simulink model "TwoArea_MA_FixedWM"  (R2020b)
settings: Solver=ode3  StartTime=0.0  StopTime=t  FixedStep=0.01  RelTol=1e-3
values from neighbouring files (symbols this model uses):
  AGC_midway = 0    [TwoAreaAGC_Parameters_Start_MA.m]    (also in result_agcimprovement.m = 1; result_replayimpact.m; result_replayimpactvaryingload.m; result_replaywithoutwm.m)
  Apc = [-par.D/(2*par.H)  1/(2*par.H)  0  -1/(2*par.H) ... (first row only)    [get_ssplant_1turb.m]
  Aq = zeros(N,N,nyp)    [offline_watermarking.m]
  attack_cont = 1    [TwoAreaAGC_Parameters_Start_MA.m]    (also in result_agcimprovement.m = 0; result_replayimpact.m; result_replayimpactvaryingload.m = 0; result_replaywithoutwm.m)
  attack_meas = 1    [TwoAreaAGC_Parameters_Start_MA.m]    (also in result_agcimprovement.m = 0; result_replayimpact.m; result_replayimpactvaryingload.m; result_replaywithoutwm.m)
  attack_start = 300    [TwoAreaAGC_Parameters_Start_MA.m]
  attack_type = 1    [TwoAreaAGC_Parameters_Start_MA.m]    (also in result_agcimprovement.m; result_replayimpact.m; result_replayimpactvaryingload.m; result_replaywithoutwm.m)
  Aw = zeros(N,N,nyp)    [offline_watermarking.m]
  Bpc = [0  -1/(2*par.H) ... (first row only)    [get_ssplant_1turb.m]
  Bq = zeros(N,1,nyp)    [offline_watermarking.m]
  Bw = zeros(N,1,nyp)    [offline_watermarking.m]
  C_sysd = c2d(C_sysc,ts_c)    [get_sscontr_2area.m]
  Cpc = [1 0 0 0 ... (first row only)    [get_ssplant_1turb.m]
  Cq = zeros(1,N,nyp)    [offline_watermarking.m]
  Cw = zeros(1,N,nyp)    [offline_watermarking.m]
  Dq = zeros(1,1,nyp)    [offline_watermarking.m]
  Dw = zeros(1,1,nyp)    [offline_watermarking.m]
  Ps = 2    [TwoAreaAGC_Parameters_Start_MA.m]
  scaling_replay = 2    [TwoAreaAGC_Parameters_Start_MA.m]    (also in result_agcimprovement.m = 1; result_replayimpact.m; result_replayimpactvaryingload.m; result_replaywithoutwm.m)
  status_load = 0    [TwoAreaAGC_Parameters_Start_MA.m]    (also in result_agcimprovement.m; result_replayimpact.m; result_replayimpactvaryingload.m = 1; result_replaywithoutwm.m)
  status_wm = 1    [TwoAreaAGC_Parameters_Start_MA.m]    (also in result_agcimprovement.m = 0; result_replayimpact.m = 0; result_replayimpactvaryingload.m = 0; result_replaywithoutwm.m = 0)
  ts = 1e-2    (= 0.01)    [TwoAreaAGC_Parameters_Start_MA.m]
undefined symbols (not defined in the file or in its folder): Ag, Ah, Bg, Bh, ca, Cg, Ch, Dg, Dh, DiscIntNeverNeededParam, Dpc, eta1, eta2, L1, L2, obs1, obs2, P1_sysd, P2_sysd, par1, par2, wm, xi1, xi2
libraries: cstblocks x16, dspsrcs4 x5, eeLuenbergerObserver x2
(part 2 of 2)

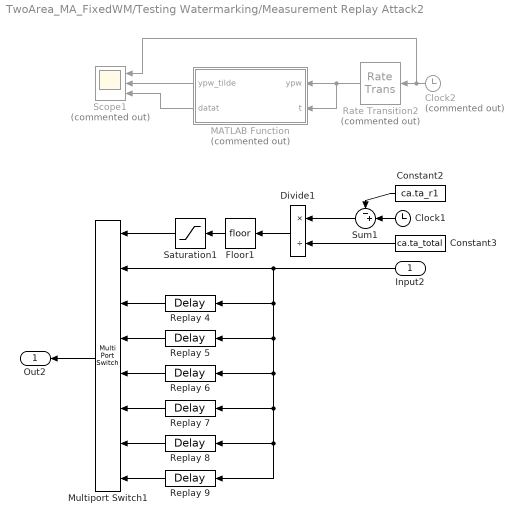
== system TwoArea_MA_FixedWM/Testing Watermarking/Measurement Replay Attack2 ==
  Input2 : Inport
  Clock1 : Clock
  Clock2 : Clock  Commented=on
  Constant2 : Constant  Value=ca.ta_r1
  Constant3 : Constant  Value=ca.ta_total
  Divide1 : Product  Inputs=*/  OutMin=0  OutMax=3  SaturateOnIntegerOverflow=on
  Floor1 : Rounding
  MATLAB Function : MATLAB Function  Commented=on  TreatAsAtomicUnit=on
  Multiport Switch1 : MultiPortSwitch  DataPortOrder=Zero-based contiguous  Inputs=7  zeroidx=on
  Rate Transition2 : RateTransition  Commented=on  OutPortSampleTime=1
  Replay 4 : TransportDelay  DelayTime=ca.ta_total
  Replay 5 : TransportDelay  DelayTime=ca.ta_total*2
  Replay 6 : TransportDelay  DelayTime=ca.ta_total*3
  Replay 7 : TransportDelay  DelayTime=ca.ta_total*4
  Replay 8 : TransportDelay  DelayTime=ca.ta_total*5
  Replay 9 : TransportDelay  DelayTime=ca.ta_total*6
  Saturation1 : Saturate  UpperLimit=6  LowerLimit=0
  Scope1 : Scope  Commented=on  NumInputPorts=3
  Sum1 : Sum  Inputs=-+|
  Out2 : Outport
  wires:
  MATLAB Function/1(ypw_tilde) -> Scope1/2
  MATLAB Function/2(datat) -> Scope1/3
  Rate Transition2/1 -> MATLAB Function/2(t), MATLAB Function/1(ypw)
  Clock2/1 -> Scope1/1, Rate Transition2/1
  Saturation1/1 -> Multiport Switch1/1
  Input2/1 -> Replay 9/1, Replay 8/1, Replay 7/1, Replay 6/1, Replay 5/1, Replay 4/1, Multiport Switch1/2
  Sum1/1 -> Divide1/1
  Replay 4/1 -> Multiport Switch1/3
  Floor1/1 -> Saturation1/1
  Replay 5/1 -> Multiport Switch1/4
  Multiport Switch1/1 -> Out2/1
  Constant3/1 -> Divide1/2
  Replay 9/1 -> Multiport Switch1/8
  Replay 8/1 -> Multiport Switch1/7
  Divide1/1 -> Floor1/1
  Replay 7/1 -> Multiport Switch1/6
  Constant2/1 -> Sum1/1
  Clock1/1 -> Sum1/2
  Replay 6/1 -> Multiport Switch1/5

== system TwoArea_MA_FixedWM/W (Watermarker)/ W selector2 ==
  Constant10 : Constant  Value=Bw  VectorParams1D=off
  Constant11 : Constant  Value=Cw  VectorParams1D=off
  Constant12 : Constant  Value=Dw  VectorParams1D=off
  Constant9 : Constant  Value=Aw  VectorParams1D=off
  Counter : Subsystem
  MATLAB Function : MATLAB Function  TreatAsAtomicUnit=on
  Aw : Outport
  Bw : Outport  Port=2
  Cw : Outport  Port=3
  Dw : Outport  Port=4
  wires:
  Constant9/1 -> MATLAB Function/2(Aa)
  Constant10/1 -> MATLAB Function/3(Ba)
  Constant11/1 -> MATLAB Function/4(Ca)
  Constant12/1 -> MATLAB Function/5(Da)
  Counter/1(WM_rotation) -> MATLAB Function/1(WM_rotation)
  MATLAB Function/4(D) -> Dw/1
  MATLAB Function/3(C) -> Cw/1
  MATLAB Function/2(B) -> Bw/1
  MATLAB Function/1(A) -> Aw/1

== system TwoArea_MA_FixedWM/W (Watermarker)/W selector 1 ==
  Constant10 : Constant  Value=Bw  VectorParams1D=off
  Constant11 : Constant  Value=Cw  VectorParams1D=off
  Constant12 : Constant  Value=Dw  VectorParams1D=off
  Constant9 : Constant  Value=Aw  VectorParams1D=off
  Counter : Subsystem
  MATLAB Function : MATLAB Function  TreatAsAtomicUnit=on
  Aw : Outport
  Bw : Outport  Port=2
  Cw : Outport  Port=3
  Dw : Outport  Port=4
  wires:
  Constant9/1 -> MATLAB Function/2(Aa)
  Constant10/1 -> MATLAB Function/3(Ba)
  Constant11/1 -> MATLAB Function/4(Ca)
  Constant12/1 -> MATLAB Function/5(Da)
  Counter/1(WM_rotation) -> MATLAB Function/1(WM_rotation)
  MATLAB Function/4(D) -> Dw/1
  MATLAB Function/3(C) -> Cw/1
  MATLAB Function/2(B) -> Bw/1
  MATLAB Function/1(A) -> Aw/1

== system TwoArea_MA_FixedWM/W (Watermarker)/W selector3 ==
  Constant10 : Constant  Value=Bw  VectorParams1D=off
  Constant11 : Constant  Value=Cw  VectorParams1D=off
  Constant12 : Constant  Value=Dw  VectorParams1D=off
  Constant9 : Constant  Value=Aw  VectorParams1D=off
  Counter : Subsystem
  MATLAB Function : MATLAB Function  TreatAsAtomicUnit=on
  Aw : Outport
  Bw : Outport  Port=2
  Cw : Outport  Port=3
  Dw : Outport  Port=4
  wires:
  Constant9/1 -> MATLAB Function/2(Aa)
  Constant10/1 -> MATLAB Function/3(Ba)
  Constant11/1 -> MATLAB Function/4(Ca)
  Constant12/1 -> MATLAB Function/5(Da)
  Counter/1(WM_rotation) -> MATLAB Function/1(WM_rotation)
  MATLAB Function/4(D) -> Dw/1
  MATLAB Function/3(C) -> Cw/1
  MATLAB Function/2(B) -> Bw/1
  MATLAB Function/1(A) -> Aw/1

== system TwoArea_MA_FixedWM/G (Watermarker)/ G selector/Counter ==
  Constant34 : Constant
  Constant35 : Constant
  Delay : Delay  DelayLength=1  SampleTime=wm.t
  Sum : Sum
  Switch : Switch  Criteria=u2 > Threshold  Threshold=3
  WM_rotation : Outport
  wires:
  Constant35/1 -> Switch/1
  Constant34/1 -> Sum/1
  Delay/1 -> Switch/2, Sum/2
  Sum/1 -> Switch/3
  Switch/1 -> WM_rotation/1, Delay/1

== system TwoArea_MA_FixedWM/G (Watermarker)/ G selector1/Counter ==
  Constant34 : Constant
  Constant35 : Constant
  Delay : Delay  DelayLength=1  SampleTime=wm.t
  Sum : Sum
  Switch : Switch  Criteria=u2 > Threshold  Threshold=3
  WM_rotation : Outport
  wires:
  Constant35/1 -> Switch/1
  Constant34/1 -> Sum/1
  Delay/1 -> Switch/2, Sum/2
  Sum/1 -> Switch/3
  Switch/1 -> WM_rotation/1, Delay/1

== system TwoArea_MA_FixedWM/H (Watermark Remover)/ H selector/Counter ==
  Constant34 : Constant
  Constant35 : Constant
  Delay : Delay  DelayLength=1  SampleTime=wm.t
  Sum : Sum
  Switch : Switch  Criteria=u2 > Threshold  Threshold=3
  WM_rotation : Outport
  wires:
  Constant35/1 -> Switch/1
  Constant34/1 -> Sum/1
  Delay/1 -> Switch/2, Sum/2
  Sum/1 -> Switch/3
  Switch/1 -> WM_rotation/1, Delay/1

== system TwoArea_MA_FixedWM/H (Watermark Remover)/ H selector1/Counter ==
  Constant34 : Constant
  Constant35 : Constant
  Delay : Delay  DelayLength=1  SampleTime=wm.t
  Sum : Sum
  Switch : Switch  Criteria=u2 > Threshold  Threshold=3
  WM_rotation : Outport
  wires:
  Constant35/1 -> Switch/1
  Constant34/1 -> Sum/1
  Delay/1 -> Switch/2, Sum/2
  Sum/1 -> Switch/3
  Switch/1 -> WM_rotation/1, Delay/1

== system TwoArea_MA_FixedWM/Q (Watermark Remover)/ Q selector/Counter ==
  Constant34 : Constant
  Constant35 : Constant
  Delay : Delay  DelayLength=1  SampleTime=wm.t
  Sum : Sum
  Switch : Switch  Criteria=u2 > Threshold  Threshold=3
  WM_rotation : Outport
  wires:
  Constant35/1 -> Switch/1
  Constant34/1 -> Sum/1
  Delay/1 -> Switch/2, Sum/2
  Sum/1 -> Switch/3
  Switch/1 -> WM_rotation/1, Delay/1

== system TwoArea_MA_FixedWM/Q (Watermark Remover)/ Q selector1/Counter ==
  Constant34 : Constant
  Constant35 : Constant
  Delay : Delay  DelayLength=1  SampleTime=wm.t
  Sum : Sum
  Switch : Switch  Criteria=u2 > Threshold  Threshold=3
  WM_rotation : Outport
  wires:
  Constant35/1 -> Switch/1
  Constant34/1 -> Sum/1
  Delay/1 -> Switch/2, Sum/2
  Sum/1 -> Switch/3
  Switch/1 -> WM_rotation/1, Delay/1

== system TwoArea_MA_FixedWM/Q (Watermark Remover)/ Q selector2/Counter ==
  Constant34 : Constant
  Constant35 : Constant
  Delay : Delay  DelayLength=1  SampleTime=wm.t
  Sum : Sum
  Switch : Switch  Criteria=u2 > Threshold  Threshold=3
  WM_rotation : Outport
  wires:
  Constant35/1 -> Switch/1
  Constant34/1 -> Sum/1
  Delay/1 -> Switch/2, Sum/2
  Sum/1 -> Switch/3
  Switch/1 -> WM_rotation/1, Delay/1

== system TwoArea_MA_FixedWM/Testing Watermarking/ G selector/Counter ==
  Constant34 : Constant
  Constant35 : Constant
  Delay : Delay  DelayLength=1  SampleTime=wm.t
  Sum : Sum
  Switch : Switch  Criteria=u2 > Threshold  Threshold=3
  WM_rotation : Outport
  wires:
  Constant35/1 -> Switch/1
  Constant34/1 -> Sum/1
  Delay/1 -> Switch/2, Sum/2
  Sum/1 -> Switch/3
  Switch/1 -> WM_rotation/1, Delay/1

== system TwoArea_MA_FixedWM/Testing Watermarking/ H selector/Counter ==
  Constant34 : Constant
  Constant35 : Constant
  Delay : Delay  DelayLength=1  SampleTime=wm.t
  Sum : Sum
  Switch : Switch  Criteria=u2 > Threshold  Threshold=3
  WM_rotation : Outport
  wires:
  Constant35/1 -> Switch/1
  Constant34/1 -> Sum/1
  Delay/1 -> Switch/2, Sum/2
  Sum/1 -> Switch/3
  Switch/1 -> WM_rotation/1, Delay/1

== system TwoArea_MA_FixedWM/Testing Watermarking/ Q selector/Counter ==
  Constant34 : Constant
  Constant35 : Constant
  Delay : Delay  DelayLength=1  SampleTime=wm.t
  Sum : Sum
  Switch : Switch  Criteria=u2 > Threshold  Threshold=3
  WM_rotation : Outport
  wires:
  Constant35/1 -> Switch/1
  Constant34/1 -> Sum/1
  Delay/1 -> Switch/2, Sum/2
  Sum/1 -> Switch/3
  Switch/1 -> WM_rotation/1, Delay/1

== system TwoArea_MA_FixedWM/Testing Watermarking/ W selector/Counter ==
  Constant34 : Constant
  Constant35 : Constant
  Delay : Delay  DelayLength=1  SampleTime=wm.t
  Sum : Sum
  Switch : Switch  Criteria=u2 > Threshold  Threshold=3
  WM_rotation : Outport
  wires:
  Constant35/1 -> Switch/1
  Constant34/1 -> Sum/1
  Delay/1 -> Switch/2, Sum/2
  Sum/1 -> Switch/3
  Switch/1 -> WM_rotation/1, Delay/1

== system TwoArea_MA_FixedWM/W (Watermarker)/ W selector2/Counter ==
  Constant34 : Constant
  Constant35 : Constant
  Delay : Delay  DelayLength=1  SampleTime=wm.t
  Sum : Sum
  Switch : Switch  Criteria=u2 > Threshold  Threshold=3
  WM_rotation : Outport
  wires:
  Constant35/1 -> Switch/1
  Constant34/1 -> Sum/1
  Delay/1 -> Switch/2, Sum/2
  Sum/1 -> Switch/3
  Switch/1 -> WM_rotation/1, Delay/1

== system TwoArea_MA_FixedWM/W (Watermarker)/W selector 1/Counter ==
  Constant34 : Constant
  Constant35 : Constant
  Delay : Delay  DelayLength=1  SampleTime=wm.t
  Sum : Sum
  Switch : Switch  Criteria=u2 > Threshold  Threshold=3
  WM_rotation : Outport
  wires:
  Constant35/1 -> Switch/1
  Constant34/1 -> Sum/1
  Delay/1 -> Switch/2, Sum/2
  Sum/1 -> Switch/3
  Switch/1 -> WM_rotation/1, Delay/1

== system TwoArea_MA_FixedWM/W (Watermarker)/W selector3/Counter ==
  Constant34 : Constant
  Constant35 : Constant
  Delay : Delay  DelayLength=1  SampleTime=wm.t
  Sum : Sum
  Switch : Switch  Criteria=u2 > Threshold  Threshold=3
  WM_rotation : Outport
  wires:
  Constant35/1 -> Switch/1
  Constant34/1 -> Sum/1
  Delay/1 -> Switch/2, Sum/2
  Sum/1 -> Switch/3
  Switch/1 -> WM_rotation/1, Delay/1

== matlab function TwoArea_MA_FixedWM/W (Watermarker)/ W selector2/MATLAB Function ==
  data: WM_rotation input; A output; Aa input; Ba input; Ca input; Da input; B output; C output; D output
function [A,B,C,D] = WM_Selector(WM_rotation,Aa,Ba,Ca,Da)
% Select the correct watermark state space matrices for the current time
A = Aa(:,:,WM_rotation);
B = Ba(:,:,WM_rotation);
C = Ca(:,:,WM_rotation);
D = Da(:,:,WM_rotation);

== matlab function TwoArea_MA_FixedWM/W (Watermarker)/W selector 1/MATLAB Function ==
  data: WM_rotation input; A output; Aa input; Ba input; Ca input; Da input; B output; C output; D output
function [A,B,C,D] = WM_Selector(WM_rotation,Aa,Ba,Ca,Da)
% Select the correct watermark state space matrices for the current time
A = Aa(:,:,WM_rotation);
B = Ba(:,:,WM_rotation);
C = Ca(:,:,WM_rotation);
D = Da(:,:,WM_rotation);

== matlab function TwoArea_MA_FixedWM/Testing Watermarking/ H selector/MATLAB Function ==
  data: WM_rotation input; A output; Aa input; Ba input; Ca input; Da input; B output; C output; D output
function [A,B,C,D] = WM_Selector(WM_rotation,Aa,Ba,Ca,Da)
% Select the correct watermark state space matrices for the current time
A = Aa(:,:,WM_rotation);
B = Ba(:,:,WM_rotation);
C = Ca(:,:,WM_rotation);
D = Da(:,:,WM_rotation);

== matlab function TwoArea_MA_FixedWM/Testing Watermarking/ G selector/MATLAB Function ==
  data: WM_rotation input; A output; Aa input; Ba input; Ca input; Da input; B output; C output; D output
function [A,B,C,D] = WM_Selector(WM_rotation,Aa,Ba,Ca,Da)
% Select the correct watermark state space matrices for the current time
A = Aa(:,:,WM_rotation);
B = Ba(:,:,WM_rotation);
C = Ca(:,:,WM_rotation);
D = Da(:,:,WM_rotation);

== matlab function TwoArea_MA_FixedWM/Testing Watermarking/ Q selector/MATLAB Function ==
  data: WM_rotation input; A output; Aa input; Ba input; Ca input; Da input; B output; C output; D output
function [A,B,C,D] = WM_Selector(WM_rotation,Aa,Ba,Ca,Da)
% Select the correct watermark state space matrices for the current time
A = Aa(:,:,WM_rotation);
B = Ba(:,:,WM_rotation);
C = Ca(:,:,WM_rotation);
D = Da(:,:,WM_rotation);

== matlab function TwoArea_MA_FixedWM/Testing Watermarking/Measurement Replay Attack2/MATLAB Function ==
  settings: updateMethod=DISCRETE  sampleTime=1
  data: ypw input; ypw_tilde output; t input; datat output
function [ypw_tilde, datat] = fcn(ypw,t)

% Time and data parameters
tr = 150;
t0 = 300;
te = 600;
data = zeros(1,te);
data(t+1) = data(t+1) + ypw;
datat = data(t+1);

if (t >= t0) && (t < t0+tr)
    ypw_tilde = data(t0-(t-t0)-2);
else
    ypw_tilde = ypw;
end

== matlab function TwoArea_MA_FixedWM/Q (Watermark Remover)/ Q selector/MATLAB Function ==
  data: WM_rotation input; A output; Aa input; Ba input; Ca input; Da input; B output; C output; D output
function [A,B,C,D] = WM_Selector(WM_rotation,Aa,Ba,Ca,Da)
% Select the correct watermark state space matrices for the current time
A = Aa(:,:,WM_rotation);
B = Ba(:,:,WM_rotation);
C = Ca(:,:,WM_rotation);
D = Da(:,:,WM_rotation);

== matlab function TwoArea_MA_FixedWM/Q (Watermark Remover)/ Q selector1/MATLAB Function ==
  data: WM_rotation input; A output; Aa input; Ba input; Ca input; Da input; B output; C output; D output
function [A,B,C,D] = WM_Selector(WM_rotation,Aa,Ba,Ca,Da)
% Select the correct watermark state space matrices for the current time
A = Aa(:,:,WM_rotation);
B = Ba(:,:,WM_rotation);
C = Ca(:,:,WM_rotation);
D = Da(:,:,WM_rotation);

== matlab function TwoArea_MA_FixedWM/Q (Watermark Remover)/ Q selector2/MATLAB Function ==
  data: WM_rotation input; A output; Aa input; Ba input; Ca input; Da input; B output; C output; D output
function [A,B,C,D] = WM_Selector(WM_rotation,Aa,Ba,Ca,Da)
% Select the correct watermark state space matrices for the current time
A = Aa(:,:,WM_rotation);
B = Ba(:,:,WM_rotation);
C = Ca(:,:,WM_rotation);
D = Da(:,:,WM_rotation);

== matlab function TwoArea_MA_FixedWM/H (Watermark Remover)/ H selector/MATLAB Function ==
  data: WM_rotation input; A output; Aa input; Ba input; Ca input; Da input; B output; C output; D output
function [A,B,C,D] = WM_Selector(WM_rotation,Aa,Ba,Ca,Da)
% Select the correct watermark state space matrices for the current time
A = Aa(:,:,WM_rotation);
B = Ba(:,:,WM_rotation);
C = Ca(:,:,WM_rotation);
D = Da(:,:,WM_rotation);

== matlab function TwoArea_MA_FixedWM/H (Watermark Remover)/ H selector1/MATLAB Function ==
  data: WM_rotation input; A output; Aa input; Ba input; Ca input; Da input; B output; C output; D output
function [A,B,C,D] = WM_Selector(WM_rotation,Aa,Ba,Ca,Da)
% Select the correct watermark state space matrices for the current time
A = Aa(:,:,WM_rotation);
B = Ba(:,:,WM_rotation);
C = Ca(:,:,WM_rotation);
D = Da(:,:,WM_rotation);

== matlab function TwoArea_MA_FixedWM/G (Watermarker)/ G selector/MATLAB Function ==
  data: WM_rotation input; A output; Aa input; Ba input; Ca input; Da input; B output; C output; D output
function [A,B,C,D] = WM_Selector(WM_rotation,Aa,Ba,Ca,Da)
% Select the correct watermark state space matrices for the current time
A = Aa(:,:,WM_rotation);
B = Ba(:,:,WM_rotation);
C = Ca(:,:,WM_rotation);
D = Da(:,:,WM_rotation);

== matlab function TwoArea_MA_FixedWM/G (Watermarker)/ G selector1/MATLAB Function ==
  data: WM_rotation input; A output; Aa input; Ba input; Ca input; Da input; B output; C output; D output
function [A,B,C,D] = WM_Selector(WM_rotation,Aa,Ba,Ca,Da)
% Select the correct watermark state space matrices for the current time
A = Aa(:,:,WM_rotation);
B = Ba(:,:,WM_rotation);
C = Ca(:,:,WM_rotation);
D = Da(:,:,WM_rotation);

== matlab function TwoArea_MA_FixedWM/Observer Area 1/MATLAB Function ==
  data: flag1 input; flag1 output; flag2 input; time input; df_r input; dPtie_r input; df1_t input; dPtie_t input; flag2 output; detections_area1_df output; detections_area1_dPtie output
function [flag1,flag2,detections_area1_df,detections_area1_dPtie] = ...
    detection_area1(flag1,flag2,time,df_r,dPtie_r,df1_t,dPtie_t)

% Detection througb df (sum zeros and first detection time)
if flag1 == 0
    if df_r >= df1_t
        detections_area1_df = time;
        flag1 = 1;
    else
        detections_area1_df = 0;
    end
else
    detections_area1_df = 0;
end

% Detection througb dPtie (sum zeros and first detection time)
if flag2 == 0
    if dPtie_r >= dPtie_t
        detections_area1_dPtie = time;
        flag2 = 1;
    else
        detections_area1_dPtie = 0;
    end
else
    detections_area1_dPtie = 0;
end

== matlab function TwoArea_MA_FixedWM/Observer Area 1/Threshold obs1 ==
  settings: updateMethod=DISCRETE  sampleTime=1
  data: k input; yr_thres1 output; alpha input; delta input; yr_thres2 output; eta_ub input; xi_ub input; xr0_ub input; K_norm input
function [yr_thres1,yr_thres2] = thres (k,alpha,delta,eta_ub,xi_ub,xr0_ub,K_norm)

% Initialize sum terms
sum1 = zeros(1,k);
sum2 = zeros(1,k);

% Summation terms
for h = 0:k-1
    sum1(h+1) = (delta(1)^(k-1-h))*(eta_ub+K_norm*xi_ub);
    sum2(h+1) = (delta(2)^(k-1-h))*(eta_ub+K_norm*xi_ub);
end    

% Thresholds
yr_thres1 = alpha(1)*(sum(sum1)+(delta(1)^k)*xr0_ub)+xi_ub;
yr_thres2 = alpha(2)*(sum(sum2)+(delta(2)^k)*xr0_ub)+xi_ub;

== matlab function TwoArea_MA_FixedWM/Testing Watermarking/Measurement Replay Attack1/MATLAB Function ==
  data: input input; output output; t input; ta_r1 input; ta_r2 input; counter input; counter output
function [output,counter] = replayattack(input,t,ta_r1,ta_r2,counter)
% Replay attack

if t < ta_r1 %no attack
    output = input;
elseif (t >= ta_r1) && (t < ta_r2) %recording
    recording(t-ta_r1) = input;
    output = recording(t-ta_r1);
elseif t >= ta_r2 %replaying
    counter = counter + 1;
else
    output = input;
end

== matlab function TwoArea_MA_FixedWM/Testing Watermarking/Measurement Replay Attack1/MATLAB Function1 ==
  settings: updateMethod=DISCRETE  sampleTime=1
  data: ypw input; ypw_tilde output; t input; datat output
function [ypw_tilde, datat] = fcn(ypw,t)

% Time and data parameters
tr = 150;
t0 = 300;
te = 600;
data = zeros(1,te);
data(t+1) = data(t+1) + ypw;
datat = data(t+1);

if (t >= t0) && (t < t0+tr)
    ypw_tilde = data(t0-(t-t0)-2);
else
    ypw_tilde = ypw;
end

== matlab function TwoArea_MA_FixedWM/Testing Watermarking/ W selector/MATLAB Function ==
  data: WM_rotation input; A output; Aa input; Ba input; Ca input; Da input; B output; C output; D output
function [A,B,C,D] = WM_Selector(WM_rotation,Aa,Ba,Ca,Da)
% Select the correct watermark state space matrices for the current time
A = Aa(:,:,WM_rotation);
B = Ba(:,:,WM_rotation);
C = Ca(:,:,WM_rotation);
D = Da(:,:,WM_rotation);

== matlab function TwoArea_MA_FixedWM/Observer Area 2/Threshold obs2 ==
  settings: updateMethod=DISCRETE  sampleTime=1
  data: k input; yr_thres1 output; alpha input; delta input; yr_thres2 output; eta_ub input; xi_ub input; xr0_ub input; K_norm input
function [yr_thres1,yr_thres2] = thres (k,alpha,delta,eta_ub,xi_ub,xr0_ub,K_norm)

% Initialize sum terms
sum1 = zeros(1,k);
sum2 = zeros(1,k);

% Summation terms
for h = 0:k-1
    sum1(h+1) = (delta(1)^(k-1-h))*(eta_ub+K_norm*xi_ub);
    sum2(h+1) = (delta(2)^(k-1-h))*(eta_ub+K_norm*xi_ub);
end    

% Thresholds
yr_thres1 = alpha(1)*(sum(sum1)+(delta(1)^k)*xr0_ub)+xi_ub;
yr_thres2 = alpha(2)*(sum(sum2)+(delta(2)^k)*xr0_ub)+xi_ub;

== matlab function TwoArea_MA_FixedWM/W (Watermarker)/W selector3/MATLAB Function ==
  data: WM_rotation input; A output; Aa input; Ba input; Ca input; Da input; B output; C output; D output
function [A,B,C,D] = WM_Selector(WM_rotation,Aa,Ba,Ca,Da)
% Select the correct watermark state space matrices for the current time
A = Aa(:,:,WM_rotation);
B = Ba(:,:,WM_rotation);
C = Ca(:,:,WM_rotation);
D = Da(:,:,WM_rotation);
